simulink model "DC_Motor_project_TET41200_2"  (R2024b)
settings: Solver=ode23tb  StartTime=0.0  StopTime=5  MaxStep=10e-6  RelTol=1e-3  EnableMultiTasking=on
values from neighbouring files (symbols this model uses):
  A = 2.5    [Other_model_parameters.m]
  c_w = 0.2    [Other_model_parameters.m]
  g = 9.81    [Other_model_parameters.m]
  i_g = 10    [Other_model_parameters.m]
  J = J_car + J_m + J_g    (= 0.50375)    [Other_model_parameters.m]
  M = 2200    [Other_model_parameters.m]
  mu_r = 0.01    [Other_model_parameters.m]
  r_w = 0.25    [Other_model_parameters.m]
  rho = 1.2    [Other_model_parameters.m]
undefined symbols (not defined in the file or in its folder): DiscIntNeverNeededParam, eea_lib, PI, reg
libraries: spsVoltageMeasurementLib x8, simulink_extras x6, spsCurrentMeasurementLib x4, spsOnDelayLib x2, spsMonostableLib x2, spsControlledCurrentSourceLib x2, spsUniversalBridgeLib x2, spsDCVoltageSourceLib x1, sps_lib x1
(part 1 of 2)
settings Model: Creator=minothi  LastModifiedBy=runde
settings SolverCC: AlgebraicLoopSolver=TrustRegion  SolverResetMethod=Robust
settings DataIOCC: LimitDataPoints=on  SaveFormat=Array  SignalLoggingSaveFormat=ModelDataLogs  ReturnWorkspaceOutputs=off
settings OptimizationCC: ExpressionDepthLimit=2147483647  InitFltsAndDblsToZero=on  LifeSpan=inf
settings DebuggingCC: SaveWithParameterizedLinksMsg=none  UnderspecifiedInitializationDetection=Classic  MergeDetectMultiDrivingBlocksExec=none  SignalResolutionControl=TryResolveAllWithWarning  SolverPrmCheckMsg=warning  MultiTaskDSMMsg=warning  MultiTaskCondExecSysMsg=none  FcnCallInpInsideContextMsg=warning  UnconnectedInputMsg=warning  UnconnectedOutputMsg=warning  UnconnectedLineMsg=warning  AllowSymbolicDim=off  StateNameClashWarn=warning  SFUnexpectedBacktrackingDiag=warning  SFNoUnconditionalDefaultTransitionDiag=warning  SFExecutionAtInitializationDiag=none  ArithmeticOperatorsInVariantConditions=warning
settings HardwareCC: ProdBitPerPointer=32  ProdBitPerSizeT=32  ProdBitPerPtrDiffT=32  ProdLargestAtomicFloat=None  ProdIntDivRoundTo=Undefined  ProdEndianess=Unspecified  ProdWordSize=32  ProdHWDeviceType=32-bit Generic
settings ModelReferenceCC: EnableRefExpFcnMdlSchedulingChecks=on  PropagateSignalLabelsOutOfModel=off
settings SFSimCC: SimUseLocalCustomCode=off  CustomCodeUndefinedFunction=UseInterfaceOnly
settings RTWCC: RTWUseLocalCustomCode=off  GPUComputeCapability=3.5
settings CodeAppCC: StateflowObjectComments=on
settings GRTTargetCC: TargetFcnLib=ansi_tfl_tmw.mat  TargetLangStandard=C89/C90 (ANSI)  CombineOutputUpdateFcns=off  GRTInterface=on
settings ConfigComp: CovMetricSettings=dw  CovSaveCumulativeToWorkspaceVar=on  CovSaveSingleToWorkspaceVar=on  CovExternalEMLEnable=off
settings SimscapeCC: SimscapeNormalizeSystem=off

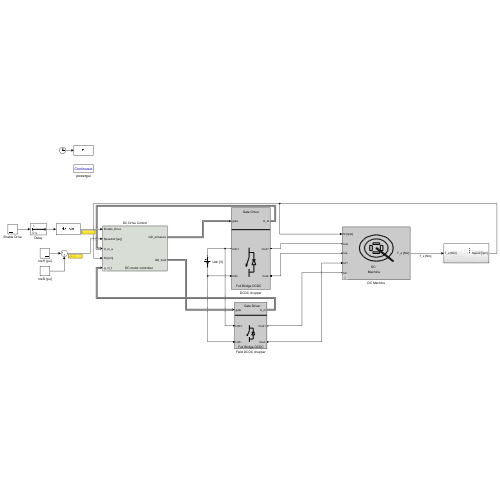
[thumbnail: Simulink's stored preview of the top-level diagram]
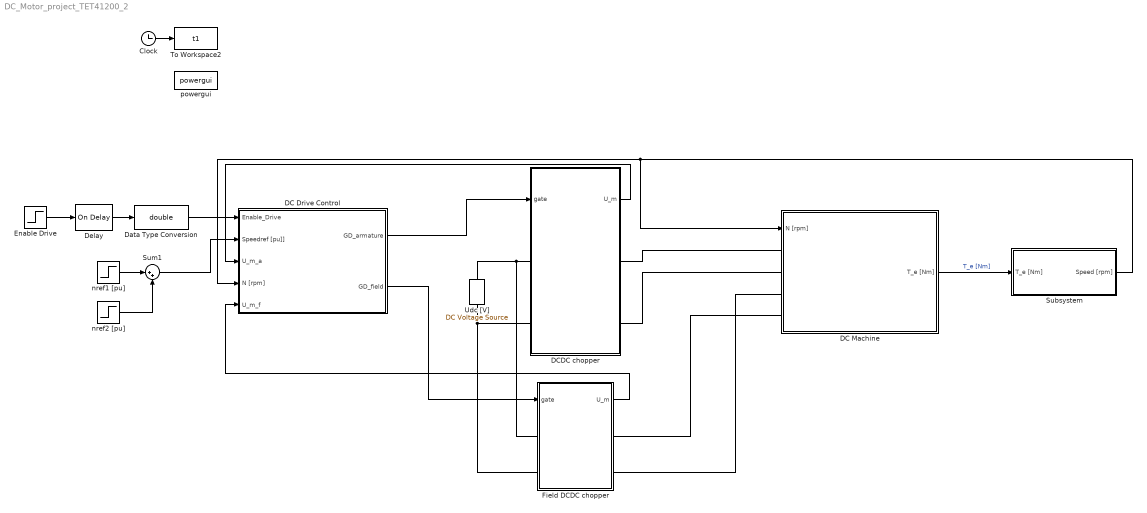
== system DC_Motor_project_TET41200_2 ==
  Clock : Clock
  DC Drive Control : Subsystem  mask{Uan=320, Ian=20, N_n=3000, Ra=1, Ufn=50, Ifn=1, I_outmax=2, I_outmin=-2, Torque_max=1.5, Torque_min=-1.5, Speed_control=1, Kp_i=0.24*1.2, Kv_i=1, Ti_i=9.75e-3, T_fa=1.0*100e-6, Kp_f=44, Ti_f=0.1, T_ff=0, Kp_n=80, Ti_n=30.8e-3, Kv_n=0, T_fn=5.5e-3, T_tri=1/1000}
      mask prompts: Uan "Uan [V]"; Ian "Ian, rated Current [A]"; N_n "Rated speed [rpm]"; Ra "Ra [Ohm]"; Ufn "Ufn [V]"; Ifn "Ifn [A]"; I_outmax "i_a,max [pu]"; I_outmin "i_a,min [pu]"; Torque_max "Torque, max [pu]"; Torque_min "Torque_min [pu]"; Speed_control "Speed control [=1. 0=Torque control]:"; Kp_i "Current controller gain K_pa"; Kv_i "Gain feedforward K__va"; Ti_i "Integration time constant T_ia"; T_fa "Armature Filter time constant T_fa [s]"; Kp_f "Field current controller gain:"; Ti_f "File Current Integration time Ti_f"; T_ff "Filter time constant field current"; Kp_n "Speed controller gain K_pn"; Ti_n "Speed Controller T_in"; Kv_n "Gain feedforward K_vn"; T_fn "Speed filter time constant"
      mask Display: text(0.350,0.08,'DC motor controller')
  DC Machine : Subsystem  mask{Uan=320, Ian=20, N_n=3000, Ra=1, La=10e-3, Ufn=50, Ifn=1, Tf=0.1}
      mask prompts: Uan "Uan, nominal Voltage [V]"; Ian "Ian, nominal current [A]"; N_n "Rated mechanical speed [rpm]"; Ra "Ra , resistance [Ohm]"; La "La,   inductance [H]"; Ufn "Ufn, nominal Field Voltage [V]"; Ifn "Ifn, nominal Field Current [A]"; Tf "Time constant field winding Tf:"
      mask Display:
      | text(0.43,0.25,'DC')
      | text(0.38,0.15,'Machine')
      | 
      | plot([0.2500    0.2600    0.2700    0.2900    0.3100    0.3300    0.3600    0.3900    0.4200    0.4600    0.5000    0.5400    0.5800    0.6100    0.6400    0.6700    0.6900    0.7100    0.7300    0.7400    0.7500], [0.6000    0.6700    0.6980    0.7356    0.7625    0.7833    0.8071    0.8245    0.8369    0.8468    0.8500    0.8468    0.8369    0.8245    0.8071    0.7833    0.7625    0.7356    0.6980    0.6700    0.6000])
      | plot([0.2500    0.2600    0.2700    0.2900    0.3100    0.3300    0.3600    0.3900    0.4200    0.4600    0.5000    0.5400    0.5800    0.6100    0.6400    0.6700    0.6900    0.7100    0.7300    0.7400    0.7500], [0.6000    0.5300    0.5020    0.4644    0.4375    0.4167    0.3929    0.3755    0.3631    0.3532    0.3500    0.3532    0.3631    0.3755    0.3929    0.4167    0.4375    0.4644    0.5020    0.5300    0.6000])
      | 
      | plot([0.3250    0.3320    0.3390    0.3530    0.3670    0.3810    0.4020    0.4230    0.4440    0.4720    0.5000    0.5280    0.5560    0.5770    0.5980    0.6190    0.6330    0.6470    0.6610    0.6680    0.6750], [0.6000    0.6490    0.6686    0.6950    0.7137    0.7283    0.7450    0.7571    0.7658    0.7727    0.7750    0.7727    0.7658    0.7571    0.7450    0.7283    0.7137    0.6950    0.6686    0.6490    0.6000])
      | plot([0.3250    0.3320    0.3390    0.3530    0.3670    0.3810    0.4020    0.4230    0.4440    0.4720    0.5000    0.5280    0.5560    0.5770    0.5980    0.6190    0.6330    0.6470    0.6610    0.6680    0.6750], [0.6000    0.5510    0.5314    0.5050    0.4863    0.4717    0.4550    0.4429    0.4342    0.4273    0.4250    0.4273    0.4342    0.4429    0.4550    0.4717    0.4863    0.5050    0.5314    0.5510    0.6000])
      | 
      | plot([0.4 0.4 0.44 0.44 0.4],   [0.55 0.65 0.65 0.55 0.55])
      | plot([0.56 0.56 0.6 0.6 0.56], [0.55 0.65 0.65 0.55 0.55])
      | plot([0.45 0.55 0.55 0.45 0.45], [0.5 0.5 0.53 0.53 0.5])
      | plot([0.45 0.55 0.55 0.45 0.45], [0.7 0.7 0.67 0.67 0.7])
      | 
      | plot([0.495 0.505 0.755 0.745 0.495], [0.595 0.605 0.355 0.345 0.595])
  DCDC chopper : Subsystem
      mask Display:
      | text(0.12,0.05,'Full Bridge DCDC')
      | text(0.3,0.95,'Gate Driver')
      | plot([0.0 1.0], [0.73 0.73])
      | plot([0.45 0.45 0.38], [0.51 0.39 0.28])
      | plot([0.45 0.45], [0.15 0.25])
      | plot([0.381 0.38 0.408], [0.317 0.28 0.302])
      | 
      | plot([0.45 0.58], [0.45 0.45])
      | plot([0.45 0.58], [0.21 0.21])
      | plot([0.58 0.58], [0.45 0.36])
      | plot([0.58 0.58], [0.21 0.30])
      | plot([0.53 0.63], [0.36 0.36])
      | plot([0.53 0.63], [0.30 0.30])
      | plot([0.53 0.58 0.63], [0.30 0.36 0.30])
  Data Type Conversion : DataTypeConversion  OutDataTypeStr=double  SaturateOnIntegerOverflow=off  RndMeth=Floor
  Delay : spsOnDelayLib/On Delay  DelayType=On delay  delay=0  ic=0  Ts=0
  Enable Drive : Step  Time=0.025  SampleTime=0
  Field DCDC chopper : Subsystem
      mask Display:
      | text(0.12,0.05,'Full Bridge DCDC')
      | text(0.3,0.95,'Gate Driver')
      | plot([0.0 1.0], [0.73 0.73])
      | plot([0.45 0.45 0.38], [0.51 0.39 0.28])
      | plot([0.45 0.45], [0.15 0.25])
      | plot([0.381 0.38 0.408], [0.317 0.28 0.302])
      | 
      | plot([0.45 0.58], [0.45 0.45])
      | plot([0.45 0.58], [0.21 0.21])
      | plot([0.58 0.58], [0.45 0.36])
      | plot([0.58 0.58], [0.21 0.30])
      | plot([0.53 0.63], [0.36 0.36])
      | plot([0.53 0.63], [0.30 0.30])
      | plot([0.53 0.58 0.63], [0.30 0.36 0.30])
  Subsystem : Subsystem
  Sum1 : Sum  Inputs=|++
  To Workspace2 : ToWorkspace  VariableName=t1  SampleTime=1e-3
  Udc [V] : spsDCVoltageSourceLib/DC Voltage Source  Amplitude=360  Measurements=None
  nref1 [pu] : Step  Time=0.2  After=-5  SampleTime=0
  nref2 [pu] : Step  Time=0.9  After=-0.1  SampleTime=0
  powergui : sps_lib/powergui  SimulationMode=Continuous  SampleTime=0  frequency=60  Iterations=50  frequencyindice=0  Pbase=100e6  ErrMax=1e-4  UnitsV=kV  UnitsW=MW  buscounter=0  FunctionMessages=off  echomessages=off  EnableUseOfTLC=off  CurrentSourceSwitches=on  DisableSnubberDevices=off  DisableRonSwitches=off  DisableVfSwitches=off  DisplayEquations=off  AutomaticDiscreteSolvers=off  SolverType=Tustin  Interpol=off  ExternalGateDelay=off  methode=off  Ts=0  x0status=blocks  SPID=off  SwTol=0  HookPort=off  NonlinearTolerance=1e-4  nMaxIteration=100  ContinueOnMaxIteration=off  RestoreLinks=warning  ResistiveCurrentMeasurement=off  Frange=[0:2:500]  Ylog=off  Xlog=on  ShowGrid=off  save=off  variable=ZData  structure=0  ZoomFFT=on  StartTime=0.0  cycles=1  DisplayStyle=1  fundamental=60  FreqAxis=off  MaxFrequency=1000  frequencyindicesteady=1  RmsSteady=1  display=off
  wires:
  Clock/1 -> To Workspace2/1
  Enable Drive/1 -> Delay/1
  DCDC chopper/1(" U_m") -> DC Drive Control/3(U_m_a)
  DC Drive Control/1(GD_armature) -> DCDC chopper/1(gate)
  Delay/1 -> Data Type Conversion/1
  Data Type Conversion/1 -> DC Drive Control/1(Enable_Drive)
  nref1 [pu]/1 -> Sum1/1
  nref2 [pu]/1 -> Sum1/2
  Sum1/1 -> DC Drive Control/2(Speedref [pu]])
  DC Drive Control/2(GD_field) -> Field DCDC chopper/1(gate)
  Field DCDC chopper/1(" U_m") -> DC Drive Control/5(U_m_f)
  Subsystem/1(Speed [rpm]) -> DC Drive Control/4(N [rpm]), DC Machine/1(N [rpm])
  DC Machine/1(T_e [Nm]) -> Subsystem/1(T_e [Nm])  "T_e [Nm]"
  connections:
  Udc [V]/RConn1 -- Field DCDC chopper/LConn1 -- DCDC chopper/LConn1
  Udc [V]/LConn1 -- DCDC chopper/LConn2 -- Field DCDC chopper/LConn2
  DC Machine/LConn1 -- DCDC chopper/RConn1
  DC Machine/LConn2 -- DCDC chopper/RConn2
  Field DCDC chopper/RConn2 -- DC Machine/LConn3
  DC Machine/LConn4 -- Field DCDC chopper/RConn1

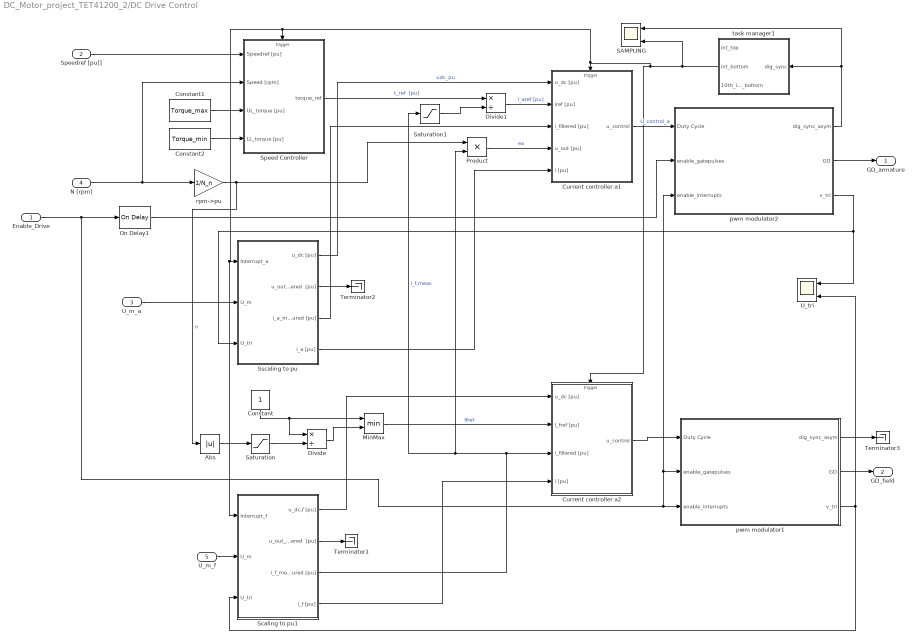
== system DC_Motor_project_TET41200_2/DC Drive Control ==
  Enable_Drive : Inport
  Speedref [pu]] : Inport  Port=2
  U_m_a : Inport  Port=3
  N [rpm] : Inport  Port=4
  U_m_f : Inport  Port=5
  Abs : Abs  SaturateOnIntegerOverflow=off
  Constant : Constant
  Constant1 : Constant  Value=Torque_max
  Constant2 : Constant  Value=Torque_min
  Current controller a1 : Subsystem
  Current controller a2 : Subsystem
  Divide : Product  Inputs=*/
  Divide1 : Product  Inputs=*/
  MinMax : MinMax  Inputs=2
  On Delay1 : spsOnDelayLib/On Delay  DelayType=On delay  delay=0  ic=0  Ts=0
  Product : Product
  SAMPLING : Scope  NumInputPorts=2
  Saturation : Saturate  UpperLimit=Inf  LowerLimit=0.01
  Saturation1 : Saturate  UpperLimit=Inf  LowerLimit=0.01
  Scaling to pu1 : Subsystem
  Speed Controller : Subsystem
  Sscaling to pu : Subsystem
  Terminator1 : Terminator
  Terminator2 : Terminator
  Terminator3 : Terminator
  U_tri : Scope  NumInputPorts=2
  pwm modulator1 : Subsystem  mask{T_tri=T_tri, t_dead=1.0e-6, t_min=3.0e-6, type_signal=1, asym=on}
      mask prompts: T_tri "Switching period  [sec]"; t_dead "t_dead, blanking time for the switches"; t_min "t_min, minimum turn off time for the swtches"; type_signal "type_signal, type of reference voltage signal (1 or 2)"; asym "Asymmetrical PWM"
      mask help:
      | The pwm module simulates a three-phase pulse-width modulator and sets the digital switch signals for six inverter switches. Nonlinear effects as blanking time and minimum turn-off time is implemented.
      |
      | As reference voltage signal can one of the following be chosen:
      | 1 - pure sinus
      | 2 - sinus with the injection of the third harmonic
      mask Display:
      | text(0.38,0.2,'DC asym pwm')
      | 
      | plot([0.32 0.32 0.68 0.68 0.32], [0.4 0.8 0.8 0.4 0.4])
      | plot([0.34 0.38 0.42 0.46 0.50 0.54 0.58 0.62 0.66], [0.5 0.7 0.5 0.7 0.5 0.7 0.5 0.7 0.5])
      | plot([0.3400    0.3600    0.3800    0.4000    0.4200    0.4400    0.4600    0.4800    0.5000    0.5200    0.5400    0.5600    0.5800    0.6000    0.6200    0.6400    0.6600], [0.6053    0.5699    0.5392    0.5182    0.5100    0.5161    0.5354    0.5650    0.6000    0.6350    0.6646    0.6839    0.6900    0.6818    0.6608    0.6301    0.5947])
  pwm modulator2 : Subsystem  mask{T_tri=T_tri, t_dead=1.0e-6, t_min=3.0e-6, type_signal=1, asym=on}
      mask prompts: T_tri "Switching period  [sec]"; t_dead "t_dead, blanking time for the switches"; t_min "t_min, minimum turn off time for the swtches"; type_signal "type_signal, type of reference voltage signal (1 or 2)"; asym "Asymmetrical PWM"
      mask help:
      | The pwm module simulates a three-phase pulse-width modulator and sets the digital switch signals for six inverter switches. Nonlinear effects as blanking time and minimum turn-off time is implemented.
      |
      | As reference voltage signal can one of the following be chosen:
      | 1 - pure sinus
      | 2 - sinus with the injection of the third harmonic
      mask Display:
      | text(0.38,0.2,'DC asym pwm')
      | 
      | plot([0.32 0.32 0.68 0.68 0.32], [0.4 0.8 0.8 0.4 0.4])
      | plot([0.34 0.38 0.42 0.46 0.50 0.54 0.58 0.62 0.66], [0.5 0.7 0.5 0.7 0.5 0.7 0.5 0.7 0.5])
      | plot([0.3400    0.3600    0.3800    0.4000    0.4200    0.4400    0.4600    0.4800    0.5000    0.5200    0.5400    0.5600    0.5800    0.6000    0.6200    0.6400    0.6600], [0.6053    0.5699    0.5392    0.5182    0.5100    0.5161    0.5354    0.5650    0.6000    0.6350    0.6646    0.6839    0.6900    0.6818    0.6608    0.6301    0.5947])
  rpm->pu : Gain  Gain=1/N_n
  task manager1 : Subsystem  mask{T_exec_0=20e-6}
      mask prompts: T_exec_0 "Execution time of Int0 (less than 0.5 T_tri)"
  GD_armature : Outport
  GD_field : Outport  Port=2
  wires:
  U_m_a/1 -> Sscaling to pu/2(U_m)
  Enable_Drive/1 -> pwm modulator1/3(enable_interrupts), pwm modulator1/2(enable_gatepulses), pwm modulator2/3(enable_interrupts), On Delay1/1
  Speed Controller/1(torque_ref) -> Divide1/1  "t_ref  [pu]"
  Sscaling to pu/3(i_a_mesured [pu]) -> Current controller a1/3(i_filtered [pu])
  Sscaling to pu/1(u_dc [pu]) -> Current controller a1/1(u_dc [pu])  "udc_pu"
  Current controller a1/1(u_control) -> pwm modulator2/1(Duty Cycle)  "U_control_a"
  N [rpm]/1 -> rpm->pu/1, Speed Controller/2(Speed [rpm])
  rpm->pu/1 -> Product/1, Abs/1  "n"
  Sscaling to pu/2(u_out_filtered  [pu]) -> Terminator2/1
  Sscaling to pu/4(i_a [pu]) -> Current controller a1/5(i [pu])
  Speedref [pu]]/1 -> Speed Controller/1(Speedref [pu])
  On Delay1/1 -> pwm modulator2/2(enable_gatepulses)
  U_m_f/1 -> Scaling to pu1/2(U_m)
  Scaling to pu1/3(i_f_mesured [pu]) -> Product/2, Saturation1/1, Current controller a2/3(i_filtered [pu])  "i_f,meas"
  Scaling to pu1/1(u_dc,f [pu]) -> Current controller a2/1(u_dc [pu])
  Constant/1 -> MinMax/1, Divide/1
  Abs/1 -> Saturation/1
  Saturation/1 -> Divide/2
  Divide/1 -> MinMax/2
  MinMax/1 -> Current controller a2/2(i_fref [pu])  "Ifref"
  Saturation1/1 -> Divide1/2
  Divide1/1 -> Current controller a1/2(iref [pu])  "i_aref [pu]"
  pwm modulator2/2(GD) -> GD_armature/1
  pwm modulator1/2(GD) -> GD_field/1
  pwm modulator2/1(dig_sync_asym) -> SAMPLING/1, task manager1/1(dig_sync)
  task manager1/2(int_bottom) -> SAMPLING/2, Current controller a2/Trigger, Speed Controller/Trigger, Scaling to pu1/1(Interrupt_f), Sscaling to pu/1(Interrupt_a), Current controller a1/Trigger
  pwm modulator1/3(v_tri) -> Scaling to pu1/3(U_tri), U_tri/2
  pwm modulator1/1(dig_sync_asym) -> Terminator3/1
  pwm modulator2/3(v_tri) -> U_tri/1, Sscaling to pu/3(U_tri)
  Current controller a2/1(u_control) -> pwm modulator1/1(Duty Cycle)
  Product/1 -> Current controller a1/4(u_out [pu])  "ea"
  Scaling to pu1/4(i_f [pu]) -> Current controller a2/4(i [pu])
  Scaling to pu1/2(u_out_filtered  [pu]) -> Terminator1/1
  Constant1/1 -> Speed Controller/3(UL_torque [pu])
  Constant2/1 -> Speed Controller/4(LL_torque [pu])

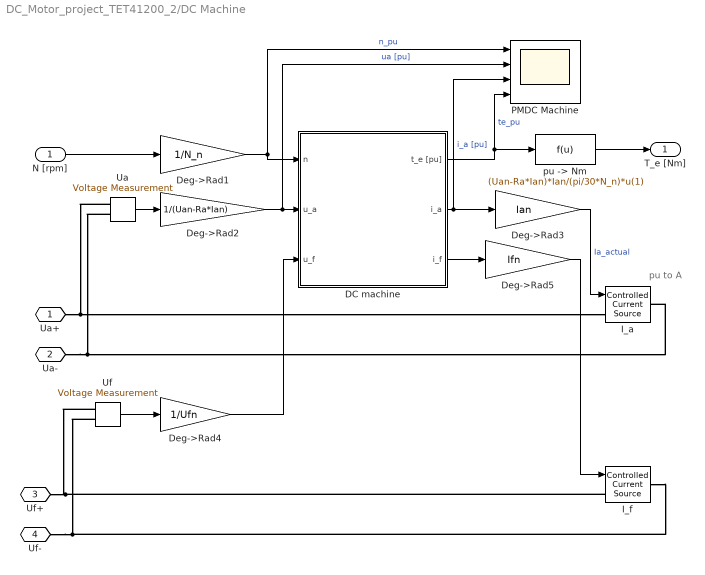
== system DC_Motor_project_TET41200_2/DC Machine ==
  note: pu to A
  N [rpm] : Inport
  DC machine : Subsystem  mask{r_a=Ra*Ian/(Uan-Ra*Ian), l_a=La*Ian/(Uan-Ra*Ian), T_f=Tf}
      mask prompts: r_a "r_a in [p.u.]"; l_a "l_a in [p.u]"; T_f "Field time constant Tf :"
      mask Display: text(0.32,0.9,'DC')
  Deg->Rad1 : Gain  Gain=1/N_n  SaturateOnIntegerOverflow=on  OutDataTypeStr=Inherit: Same as input  ParamDataTypeStr=Inherit: Same as input
  Deg->Rad2 : Gain  Gain=1/(Uan-Ra*Ian)  SaturateOnIntegerOverflow=on  OutDataTypeStr=Inherit: Same as input  ParamDataTypeStr=Inherit: Same as input
  Deg->Rad3 : Gain  Gain=Ian  SaturateOnIntegerOverflow=on  OutDataTypeStr=Inherit: Same as input  ParamDataTypeStr=Inherit: Same as input
  Deg->Rad4 : Gain  Gain=1/Ufn  SaturateOnIntegerOverflow=on  OutDataTypeStr=Inherit: Same as input  ParamDataTypeStr=Inherit: Same as input
  Deg->Rad5 : Gain  Gain=Ifn  SaturateOnIntegerOverflow=on  OutDataTypeStr=Inherit: Same as input  ParamDataTypeStr=Inherit: Same as input
  I_a : spsControlledCurrentSourceLib/Controlled Current Source  Initialize=on  Source_Type=AC  Amplitude=0  Phase=0  Frequency=0  Measurements=None
  I_f : spsControlledCurrentSourceLib/Controlled Current Source  Initialize=on  Source_Type=AC  Amplitude=0  Phase=0  Frequency=0  Measurements=None
  PMDC Machine : Scope  NumInputPorts=4
  Ua : spsVoltageMeasurementLib/Voltage Measurement  PhasorSimulation=off  OutputType=Complex  PSBequivalent=0
  Uf : spsVoltageMeasurementLib/Voltage Measurement  PhasorSimulation=off  OutputType=Complex  PSBequivalent=0
  "pu -> Nm" : Fcn  Expr=(Uan-Ra*Ian)*Ian/(pi/30*N_n)*u(1)
  Ua+ : PMIOPort  Side=Left
  Ua- : PMIOPort  Port=2  Side=Left
  Uf+ : PMIOPort  Port=3  Side=Left
  Uf- : PMIOPort  Port=4  Side=Left
  T_e [Nm] : Outport  InitialOutput=0
  wires:
  Deg->Rad2/1 -> PMDC Machine/2, DC machine/2(u_a)  "ua [pu]"
  Deg->Rad3/1 -> I_a/1  "Ia_actual"
  DC machine/2(i_a) -> Deg->Rad3/1, PMDC Machine/3  "i_a [pu]"
  Deg->Rad1/1 -> PMDC Machine/1, DC machine/1(n)  "n_pu"
  N [rpm]/1 -> Deg->Rad1/1
  Ua/1 -> Deg->Rad2/1
  "pu -> Nm"/1 -> T_e [Nm]/1
  DC machine/1(t_e [pu]) -> PMDC Machine/4, "pu -> Nm"/1  "te_pu"
  Uf/1 -> Deg->Rad4/1
  Deg->Rad4/1 -> DC machine/3(u_f)
  DC machine/3(i_f) -> Deg->Rad5/1
  Deg->Rad5/1 -> I_f/1
  connections:
  Ua-/RConn1 -- Ua/LConn2 -- I_a/RConn1
  Ua+/RConn1 -- Ua/LConn1 -- I_a/LConn1
  Uf/LConn1 -- I_f/LConn1 -- Uf+/RConn1
  Uf/LConn2 -- I_f/RConn1 -- Uf-/RConn1

== system DC_Motor_project_TET41200_2/DCDC chopper ==
  gate : Inport
  Armarture Converter currents : Scope  NumInputPorts=2
  Armarture Converter currents1 : Scope  NumInputPorts=2
  Demux : Demux  Outputs=2
  Idc : spsCurrentMeasurementLib/Current Measurement  PhasorSimulation=off  OutputType=Complex  PSBequivalent=0
  Iout : spsCurrentMeasurementLib/Current Measurement  PhasorSimulation=off  OutputType=Complex  PSBequivalent=0
  Universal Bridge : spsUniversalBridgeLib/Universal Bridge  Arms=2  SnubberResistance=1e5  SnubberCapacitance=inf  Device=MOSFET / Diodes  Ron=1e-3  Lon=0  ForwardVoltages="[  0  0  ]"  ForwardVoltage=0  GTOparameters=[ 10e-6 , 20e-6 ]  IGBTparameters=[ 1e-6 , 2e-6 ]  Measurements=All voltages and currents  Measurements_2=None  converterType=Rectifier
  u_m : Subsystem
  Udc+ : PMIOPort  Side=Left
  Udc- : PMIOPort  Port=2  Side=Left
  Vout+ : PMIOPort  Port=3  Side=Right
  Vout- : PMIOPort  Port=4  Side=Right
  " U_m" : Outport
  wires:
  u_m/1(U) -> " U_m"/1
  gate/1 -> Demux/1, Universal Bridge/1
  Iout/1 -> Armarture Converter currents/1, u_m/1(Ia)  "I_Out [A]"
  Idc/1 -> Armarture Converter currents/2  "i_DC [A]"
  Demux/2 -> Armarture Converter currents1/2
  Demux/1 -> Armarture Converter currents1/1
  connections:
  Universal Bridge/LConn1 -- Iout/LConn1
  Idc/LConn1 -- Udc+/RConn1
  Udc-/RConn1 -- u_m/LConn2 -- Universal Bridge/RConn2
  Universal Bridge/RConn1 -- u_m/LConn1 -- Idc/RConn1
  Vout+/RConn1 -- Iout/RConn1
  u_m/LConn4 -- Universal Bridge/LConn2 -- u_m/LConn3 -- Vout-/RConn1

== system DC_Motor_project_TET41200_2/Field DCDC chopper ==
  gate : Inport
  Field Converter currents : Scope  NumInputPorts=2
  Idc : spsCurrentMeasurementLib/Current Measurement  PhasorSimulation=off  OutputType=Complex  PSBequivalent=0
  Iout : spsCurrentMeasurementLib/Current Measurement  PhasorSimulation=off  OutputType=Complex  PSBequivalent=0
  Universal Bridge : spsUniversalBridgeLib/Universal Bridge  Arms=2  SnubberResistance=1e5  SnubberCapacitance=inf  Device=MOSFET / Diodes  Ron=1e-3  Lon=0  ForwardVoltages="[  0  0  ]"  ForwardVoltage=0  GTOparameters=[ 10e-6 , 20e-6 ]  IGBTparameters=[ 1e-6 , 2e-6 ]  Measurements=All voltages and currents  Measurements_2=None  converterType=Rectifier
  u_m : Subsystem
  Udc+ : PMIOPort  Side=Left
  Udc- : PMIOPort  Port=2  Side=Left
  Vout+ : PMIOPort  Port=3  Side=Right
  Vout- : PMIOPort  Port=4  Side=Right
  " U_m" : Outport
  wires:
  u_m/1(U) -> " U_m"/1
  gate/1 -> Universal Bridge/1
  Iout/1 -> Field Converter currents/1, u_m/1(Ia)  "I_Out [A]"
  Idc/1 -> Field Converter currents/2  "i_DC [A]"
  connections:
  Vout-/RConn1 -- Universal Bridge/LConn2 -- u_m/LConn4
  Idc/LConn1 -- Udc+/RConn1
  Udc-/RConn1 -- u_m/LConn2 -- Universal Bridge/RConn2
  Universal Bridge/RConn1 -- u_m/LConn1 -- Idc/RConn1
  Vout+/RConn1 -- Iout/RConn1
  Universal Bridge/LConn1 -- Iout/LConn1 -- u_m/LConn3

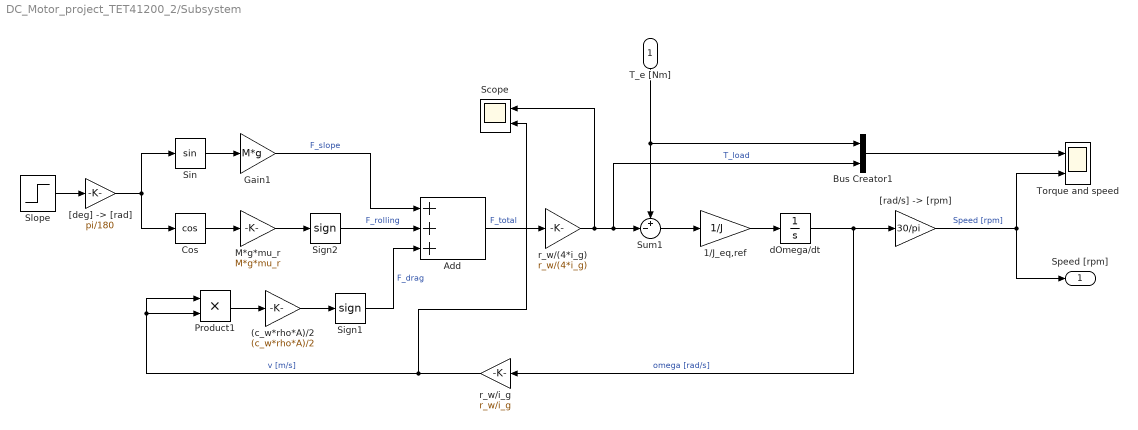
== system DC_Motor_project_TET41200_2/Subsystem ==
  T_e [Nm] : Inport
  (c_w*rho*A)/2 : Gain  Gain=(c_w*rho*A)/2
  1/J_eq,ref : Gain  Gain=1/J
  Add : Sum  Inputs=+++
  Bus Creator1 : BusCreator  Inputs=2
  Cos : Trigonometry  Operator=cos
  Gain1 : Gain  Gain=M*g
  M*g*mu_r : Gain  Gain=M*g*mu_r
  Product1 : Product
  Scope : Scope  NumInputPorts=2
  Sign1 : Signum
  Sign2 : Signum
  Sin : Trigonometry
  Slope : Step  Time=0.4  After=0  SampleTime=0
  Sum1 : Sum  Inputs=+-|
  Torque and speed : Scope  NumInputPorts=2
  "[deg] -> [rad]" : Gain  Gain=pi/180
  "[rad/s] -> [rpm]" : Gain  Gain=30/pi
  dOmega/dt : Integrator
  r_w/(4*i_g) : Gain  Gain=r_w/(4*i_g)
  r_w/i_g : Gain  Gain=r_w/i_g
  Speed [rpm] : Outport
  wires:
  Add/1 -> r_w/(4*i_g)/1  "F_total"
  1/J_eq,ref/1 -> dOmega/dt/1
  T_e [Nm]/1 -> Sum1/1, Bus Creator1/1
  Sin/1 -> Gain1/1
  Slope/1 -> "[deg] -> [rad]"/1
  Sign1/1 -> Add/3  "F_drag"
  Gain1/1 -> Add/1  "F_slope"
  Product1/1 -> (c_w*rho*A)/2/1
  r_w/(4*i_g)/1 -> Scope/1, Bus Creator1/2, Sum1/2  "T_load"
  Sign2/1 -> Add/2  "F_rolling"
  Bus Creator1/1 -> Torque and speed/1
  M*g*mu_r/1 -> Sign2/1
  Cos/1 -> M*g*mu_r/1
  Sum1/1 -> 1/J_eq,ref/1
  r_w/i_g/1 -> Scope/2, Product1/1, Product1/2  "v [m/s]"
  "[rad/s] -> [rpm]"/1 -> Speed [rpm]/1, Torque and speed/2  "Speed [rpm]"
  (c_w*rho*A)/2/1 -> Sign1/1
  dOmega/dt/1 -> "[rad/s] -> [rpm]"/1, r_w/i_g/1  "omega [rad/s]"
  "[deg] -> [rad]"/1 -> Sin/1, Cos/1

== system DC_Motor_project_TET41200_2/DC Drive Control/Current controller a1 ==
  u_dc [pu] : Inport
  iref [pu] : Inport  Port=2
  i_filtered [pu] : Inport  Port=3
  u_out [pu] : Inport  Port=4
  i [pu] : Inport  Port=5
  Trigger : TriggerPort  VariantControl=Variant
  "Armature Current Controller " : Scope  NumInputPorts=2
  Bus Creator : BusCreator  Inputs=3
  Constant : Constant
  Constant1 : Constant  Value=-1
  Current controller a : Subsystem  AncestorBlock=eea_lib/PI-reg  TreatAsAtomicUnit=on  mask{Kp=0.03, Kv=Kv_i, Ti=Ti_i, Tsamp=T_tri/2}
      mask Display:
      | text(0.32,0.05,'Digital PI-controller')
      | plot([0.2 0.8], [0.1 0.1])
      | plot([0.2 0.2], [0.1 0.9])
      | plot([0.75 0.8 0.75], [0.15 0.1 0.05])
      | plot([0.175 0.2 0.225], [0.79 0.9 0.79])
      | 
      | plot([0.2 0.75], [0.3 0.7])
  Sum : Sum  Inputs=|+-
  u_control : Outport
  wires:
  Constant1/1 -> Current controller a/5(LL)
  u_out [pu]/1 -> Current controller a/3(back_emf), Current controller a/6(Initival)
  Constant/1 -> Current controller a/4(UL)
  Sum/1 -> Current controller a/2(e)
  Bus Creator/1 -> "Armature Current Controller "/1
  Current controller a/1(Out) -> "Armature Current Controller "/2, u_control/1  "u_control"
  i [pu]/1 -> Bus Creator/3  "i_a [pu]"
  iref [pu]/1 -> Sum/1, Bus Creator/1  "i_aref [pu]"
  u_dc [pu]/1 -> Current controller a/1(gain)
  i_filtered [pu]/1 -> Bus Creator/2, Sum/2  "i_a_filtered [pu]"

== system DC_Motor_project_TET41200_2/DC Drive Control/Current controller a2 ==
  u_dc [pu] : Inport
  i_fref [pu] : Inport  Port=2
  i_filtered [pu] : Inport  Port=3
  i [pu] : Inport  Port=4
  Trigger : TriggerPort  VariantControl=Variant
  Bus Creator : BusCreator  Inputs=3
  Constant : Constant  Value=1.0
  Constant1 : Constant  Value=-1.0
  Current controller f : Subsystem  AncestorBlock=eea_lib/PI-reg  TreatAsAtomicUnit=on  mask{Kp=100, Kv=0, Ti=Ti_f, Tsamp=T_tri/2}
      mask Display:
      | text(0.32,0.05,'Digital PI-controller')
      | plot([0.2 0.8], [0.1 0.1])
      | plot([0.2 0.2], [0.1 0.9])
      | plot([0.75 0.8 0.75], [0.15 0.1 0.05])
      | plot([0.175 0.2 0.225], [0.79 0.9 0.79])
      | 
      | plot([0.2 0.75], [0.3 0.7])
  "Field Current Controller " : Scope  NumInputPorts=2
  Sum : Sum  Inputs=|+-
  u_control : Outport
  wires:
  Constant1/1 -> Current controller f/4(LL)
  Constant/1 -> Current controller f/3(UL)
  Sum/1 -> Current controller f/2(e)
  Bus Creator/1 -> "Field Current Controller "/1
  Current controller f/1(Out) -> "Field Current Controller "/2, u_control/1  "u_control_f"
  i [pu]/1 -> Bus Creator/3  "i_f [pu]"
  i_fref [pu]/1 -> Bus Creator/1, Sum/1  "i_fref [pu]"
  u_dc [pu]/1 -> Current controller f/1(gain)
  i_filtered [pu]/1 -> Sum/2, Bus Creator/2  "i_f_filtered [pu]"

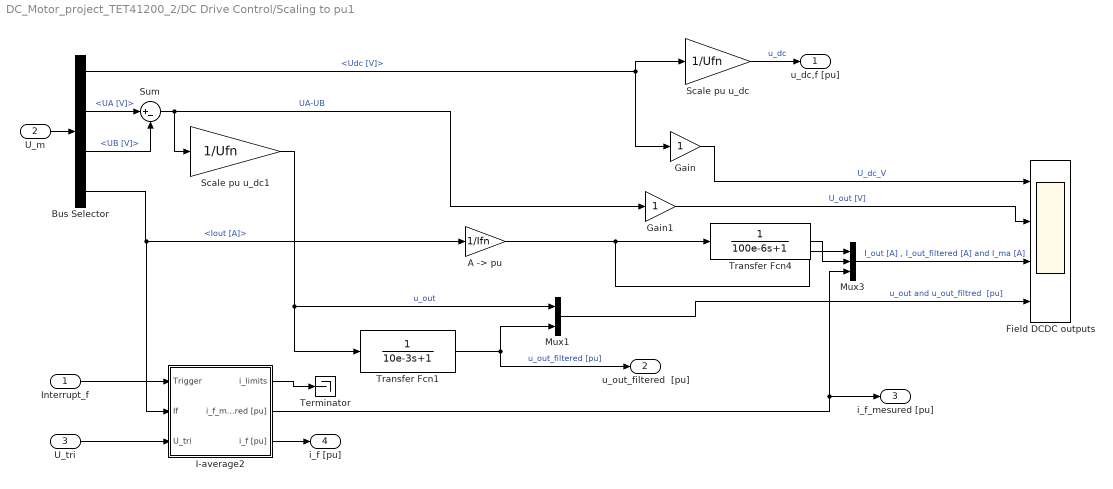
== system DC_Motor_project_TET41200_2/DC Drive Control/Scaling to pu1 ==
  Interrupt_f : Inport
  U_m : Inport  Port=2
  U_tri : Inport  Port=3
  "A -> pu" : Gain  Gain=1/Ifn
  Bus Selector : BusSelector  OutputSignals=Udc [V],UA [V],UB [V],Iout [A]
  Field DCDC outputs : Scope  NumInputPorts=4
  Gain : Gain
  Gain1 : Gain
  I-average2 : Subsystem  mask{Tsamp=T_tri/2}
  Mux1 : Mux  Inputs=2
  Mux3 : Mux  Inputs=3
  Scale pu u_dc : Gain  Gain=1/Ufn
  Scale pu u_dc1 : Gain  Gain=1/Ufn
  Sum : Sum  Inputs=|+-
  Terminator : Terminator
  Transfer Fcn1 : TransferFcn  Denominator=[10e-3 1]
  Transfer Fcn4 : TransferFcn  Denominator=[100e-6 1]
  u_dc,f [pu] : Outport
  u_out_filtered  [pu] : Outport  Port=2
  i_f_mesured [pu] : Outport  Port=3
  i_f [pu] : Outport  Port=4
  wires:
  Scale pu u_dc/1 -> u_dc,f [pu]/1  "u_dc"
  U_m/1 -> Bus Selector/1
  Scale pu u_dc1/1 -> Transfer Fcn1/1, Mux1/1  "u_out"
  Bus Selector/1 -> Scale pu u_dc/1, Gain/1  "<Udc [V]>"
  Gain/1 -> Field DCDC outputs/1  "U_dc_V"
  Bus Selector/2 -> Sum/1  "<UA [V]>"
  Gain1/1 -> Field DCDC outputs/2  "U_out [V]"
  Bus Selector/4 -> "A -> pu"/1, I-average2/2(If)  "<Iout [A]>"
  Transfer Fcn1/1 -> Mux1/2, u_out_filtered  [pu]/1  "u_out_filtered [pu]"
  Mux1/1 -> Field DCDC outputs/4  "u_out and u_out_filtred  [pu]"
  Transfer Fcn4/1 -> Mux3/2
  Mux3/1 -> Field DCDC outputs/3  "I_out [A] , I_out_filtered [A] and I_ma [A]"
  Interrupt_f/1 -> I-average2/1(Trigger)
  I-average2/2(i_f_measured [pu]) -> i_f_mesured [pu]/1, Mux3/3
  I-average2/1(i_limits) -> Terminator/1
  Bus Selector/3 -> Sum/2  "<UB [V]>"
  Sum/1 -> Scale pu u_dc1/1, Gain1/1  "UA-UB"
  I-average2/3(i_f [pu]) -> i_f [pu]/1
  U_tri/1 -> I-average2/3(U_tri)
  "A -> pu"/1 -> Transfer Fcn4/1, Mux3/1

== system DC_Motor_project_TET41200_2/DC Drive Control/Speed Controller ==
  Speedref [pu] : Inport
  Speed [rpm] : Inport  Port=2
  UL_torque [pu] : Inport  Port=3
  LL_torque [pu] : Inport  Port=4
  Trigger : TriggerPort  VariantControl=Variant
  1st order Discrete Filter : DiscreteFilter  Numerator=[T_tri/(2*T_fn)]  Denominator=[1 -(1-T_tri/(2*T_fn))]
  Bus Creator : BusCreator  Inputs=3
  "Speed Controller Controller " : Scope  NumInputPorts=3
  "Speed controller " : Subsystem  AncestorBlock=eea_lib/PI-reg  TreatAsAtomicUnit=on  mask{Kp=Kp_n, Kv=Kv_n, Ti=Ti_n, Tsamp=T_tri/2}
      mask Display:
      | text(0.32,0.05,'Digital PI-controller')
      | plot([0.2 0.8], [0.1 0.1])
      | plot([0.2 0.2], [0.1 0.9])
      | plot([0.75 0.8 0.75], [0.15 0.1 0.05])
      | plot([0.175 0.2 0.225], [0.79 0.9 0.79])
      | 
      | plot([0.2 0.75], [0.3 0.7])
  Sum : Sum  Inputs=|+-
  rpm->pu : Gain  Gain=1/N_n
  torque_ref : Outport
  wires:
  Sum/1 -> "Speed controller "/1(e), "Speed Controller Controller "/2  "n_ref - n_filtered [pu]"
  Speedref [pu]/1 -> Sum/1, Bus Creator/1  "n_ref [pu]"
  rpm->pu/1 -> 1st order Discrete Filter/1, Sum/2, Bus Creator/3  "n  [pu]"
  Speed [rpm]/1 -> rpm->pu/1
  Bus Creator/1 -> "Speed Controller Controller "/1
  "Speed controller "/1(Out) -> "Speed Controller Controller "/3, torque_ref/1
  UL_torque [pu]/1 -> "Speed controller "/2(UL)
  LL_torque [pu]/1 -> "Speed controller "/3(LL)
  1st order Discrete Filter/1 -> Bus Creator/2  "n_filtered [pu]"

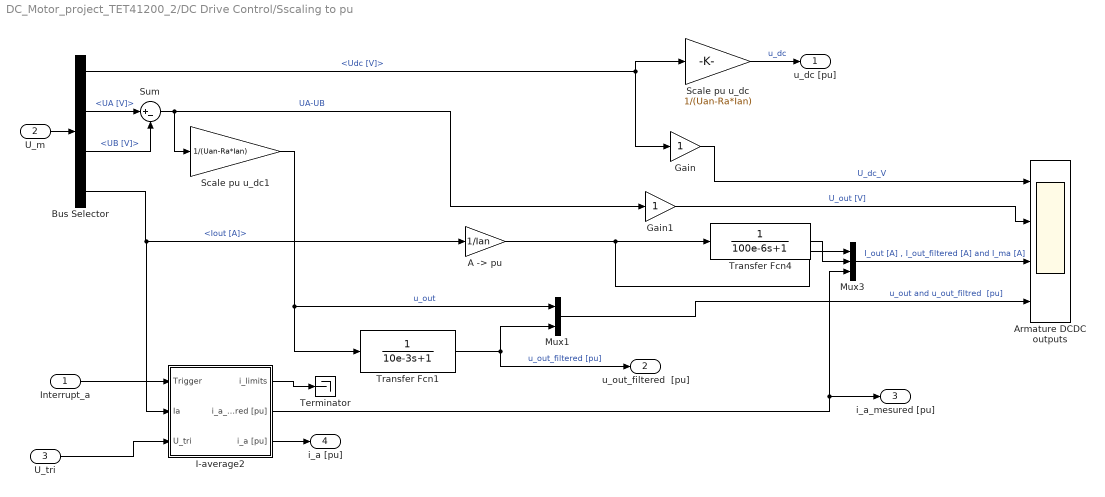
== system DC_Motor_project_TET41200_2/DC Drive Control/Sscaling to pu ==
  Interrupt_a : Inport
  U_m : Inport  Port=2
  U_tri : Inport  Port=3
  "A -> pu" : Gain  Gain=1/Ian
  Armature DCDC outputs : Scope  NumInputPorts=4
  Bus Selector : BusSelector  OutputSignals=Udc [V],UA [V],UB [V],Iout [A]
  Gain : Gain
  Gain1 : Gain
  I-average2 : Subsystem  mask{Tsamp=T_tri/2}
  Mux1 : Mux  Inputs=2
  Mux3 : Mux  Inputs=3
  Scale pu u_dc : Gain  Gain=1/(Uan-Ra*Ian)
  Scale pu u_dc1 : Gain  Gain=1/(Uan-Ra*Ian)
  Sum : Sum  Inputs=|+-
  Terminator : Terminator
  Transfer Fcn1 : TransferFcn  Denominator=[10e-3 1]
  Transfer Fcn4 : TransferFcn  Denominator=[100e-6 1]
  u_dc [pu] : Outport
  u_out_filtered  [pu] : Outport  Port=2
  i_a_mesured [pu] : Outport  Port=3
  i_a [pu] : Outport  Port=4
  wires:
  Scale pu u_dc/1 -> u_dc [pu]/1  "u_dc"
  U_m/1 -> Bus Selector/1
  Scale pu u_dc1/1 -> Transfer Fcn1/1, Mux1/1  "u_out"
  Bus Selector/1 -> Scale pu u_dc/1, Gain/1  "<Udc [V]>"
  Gain/1 -> Armature DCDC outputs/1  "U_dc_V"
  Bus Selector/2 -> Sum/1  "<UA [V]>"
  Gain1/1 -> Armature DCDC outputs/2  "U_out [V]"
  Bus Selector/4 -> "A -> pu"/1, I-average2/2(Ia)  "<Iout [A]>"
  Transfer Fcn1/1 -> Mux1/2, u_out_filtered  [pu]/1  "u_out_filtered [pu]"
  Mux1/1 -> Armature DCDC outputs/4  "u_out and u_out_filtred  [pu]"
  Transfer Fcn4/1 -> Mux3/2
  Mux3/1 -> Armature DCDC outputs/3  "I_out [A] , I_out_filtered [A] and I_ma [A]"
  Interrupt_a/1 -> I-average2/1(Trigger)
  I-average2/2(i_a_measured [pu]) -> i_a_mesured [pu]/1, Mux3/3
  I-average2/1(i_limits) -> Terminator/1
  Bus Selector/3 -> Sum/2  "<UB [V]>"
  Sum/1 -> Scale pu u_dc1/1, Gain1/1  "UA-UB"
  I-average2/3(i_a [pu]) -> i_a [pu]/1
  U_tri/1 -> I-average2/3(U_tri)
  "A -> pu"/1 -> Transfer Fcn4/1, Mux3/1

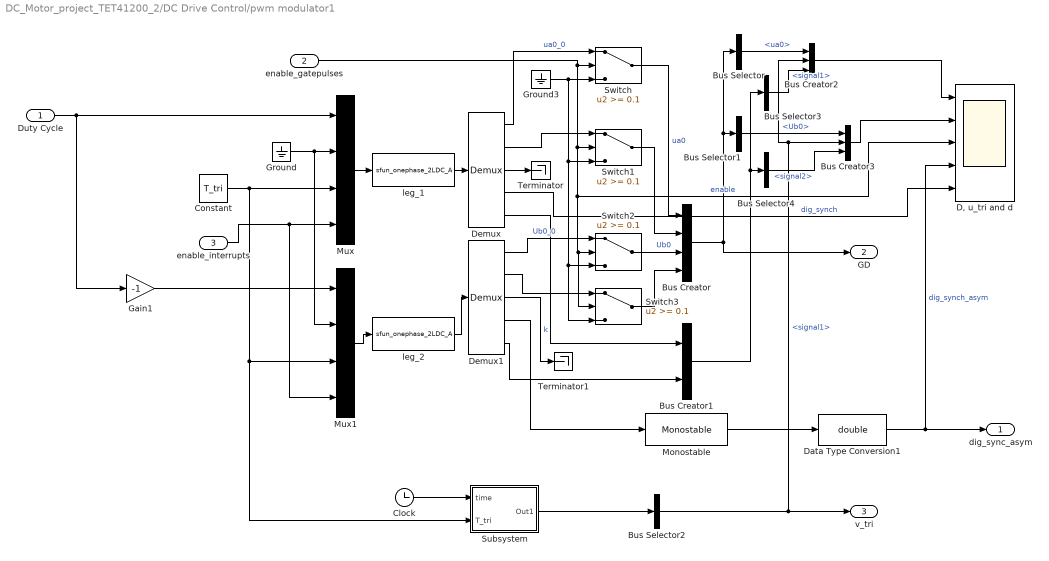
== system DC_Motor_project_TET41200_2/DC Drive Control/pwm modulator1 ==
  Duty Cycle : Inport
  enable_gatepulses : Inport  Port=2
  enable_interrupts : Inport  Port=3
  Bus Creator : BusCreator  Inputs=4
  Bus Creator1 : BusCreator  Inputs=2
  Bus Creator2 : BusCreator  Inputs=3
  Bus Creator3 : BusCreator  Inputs=3
  Bus Selector : BusSelector  OutputSignals=ua0
  Bus Selector1 : BusSelector  OutputSignals=Ub0
  Bus Selector2 : BusSelector  OutputSignals=signal1
  Bus Selector3 : BusSelector  OutputSignals=signal1
  Bus Selector4 : BusSelector  OutputSignals=signal2
  Clock : Clock
  Constant : Constant  Value=T_tri
  "D, u_tri and d " : Scope  NumInputPorts=5
  Data Type Conversion1 : DataTypeConversion  OutDataTypeStr=double  SaturateOnIntegerOverflow=off  RndMeth=Floor
  Demux : Demux  Outputs=5
      settings: DisplayOption=none
  Demux1 : Demux  Outputs=5
      settings: DisplayOption=none
  Gain1 : Gain  Gain=-1
  Ground : Ground
  Ground3 : Ground
  Monostable : spsMonostableLib/Monostable  EdgeDetect=Either  PulseDuration=T_tri/4  ic=0  Ts=0
      settings: LibrarySourceBlock=sps_lib/Control/Monostable
  Mux : Mux
  Mux1 : Mux
  Subsystem : Subsystem
  Switch{,1..3} (4 alike) : Switch  Threshold=0.1  SaturateOnIntegerOverflow=off  InputSameDT=off
  Terminator : Terminator
  Terminator1 : Terminator
  leg_1 : S-Function  FunctionName=sfun_onephase_2LDC_A  Parameters=0,t_dead,t_min,type_signal,asym  SFunctionDeploymentMode=off  EnableBusSupport=off
  leg_2 : S-Function  FunctionName=sfun_onephase_2LDC_A  Parameters=0,t_dead,t_min,type_signal,asym  SFunctionDeploymentMode=off  EnableBusSupport=off
  dig_sync_asym : Outport
  GD : Outport  Port=2
  v_tri : Outport  Port=3
  wires:
  Demux/3 -> Terminator/1
  Constant/1 -> Mux/3, Subsystem/2(T_tri), Mux1/3
  Ground/1 -> Mux1/2, Mux/2
  leg_1/1 -> Demux/1
  leg_2/1 -> Demux1/1
  Mux/1 -> leg_1/1
  Demux/2 -> Switch1/1
  Demux1/5 -> Bus Creator1/2
  Demux/4 -> "D, u_tri and d "/5  "dig_synch"
  Subsystem/1(Out1) -> Bus Selector2/1
  Clock/1 -> Subsystem/1(time)
  Demux/5 -> Bus Creator1/1
  Bus Creator/1 -> GD/1, Bus Selector1/1, Bus Selector/1
  Bus Creator1/1 -> Bus Selector3/1, Bus Selector4/1
  Bus Selector/1 -> Bus Creator2/1  "<ua0>"
  Bus Selector3/1 -> Bus Creator2/3  "<signal1>"
  Bus Selector1/1 -> Bus Creator3/1  "<Ub0>"
  Bus Selector4/1 -> Bus Creator3/3  "<signal2>"
  Bus Creator2/1 -> "D, u_tri and d "/1
  Bus Creator3/1 -> "D, u_tri and d "/2
  Mux1/1 -> leg_2/1
  enable_gatepulses/1 -> Switch/2, Switch3/2, Switch2/2, "D, u_tri and d "/3, Switch1/2  "enable"
  Duty Cycle/1 -> Mux/1, Gain1/1
  Gain1/1 -> Mux1/1
  Switch/1 -> Bus Creator/1  "ua0"
  Demux/1 -> Switch/1  "ua0_0"
  Switch1/1 -> Bus Creator/2
  Ground3/1 -> Switch/3, Switch1/3, Switch2/3, Switch3/3
  Switch2/1 -> Bus Creator/3  "Ub0"
  Switch3/1 -> Bus Creator/4
  Bus Selector2/1 -> Bus Creator2/2, Bus Creator3/2, v_tri/1  "<signal1>"
  Demux1/4 -> Monostable/1
  Monostable/1 -> Data Type Conversion1/1
  Data Type Conversion1/1 -> dig_sync_asym/1, "D, u_tri and d "/4  "dig_synch_asym"
  Demux1/3 -> Terminator1/1  "k"
  enable_interrupts/1 -> Mux1/4, Mux/4
  Demux1/1 -> Switch2/1  "Ub0_0"
  Demux1/2 -> Switch3/1

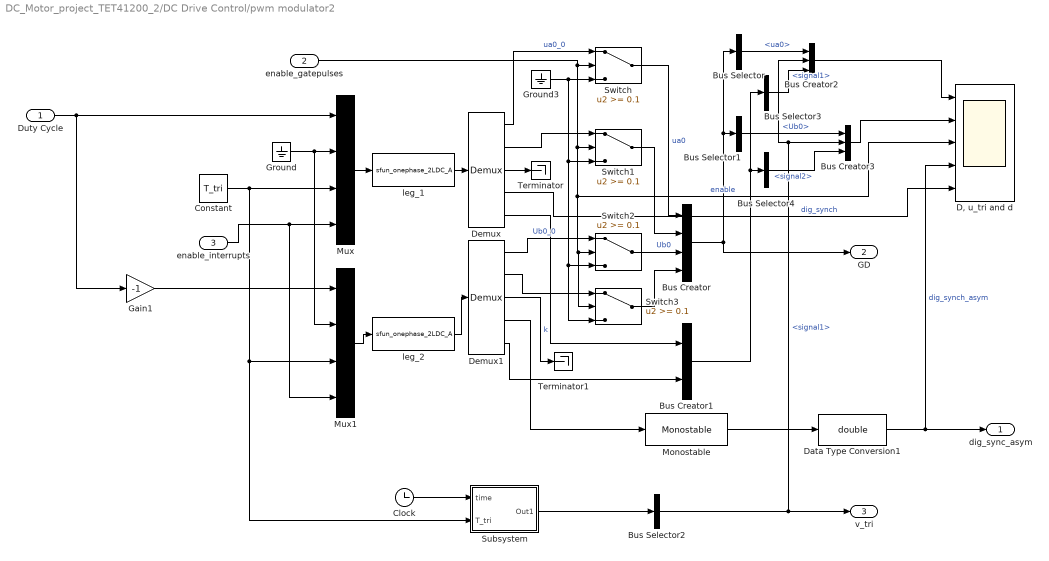
== system DC_Motor_project_TET41200_2/DC Drive Control/pwm modulator2 ==
  Duty Cycle : Inport
  enable_gatepulses : Inport  Port=2
  enable_interrupts : Inport  Port=3
  Bus Creator : BusCreator  Inputs=4
  Bus Creator1 : BusCreator  Inputs=2
  Bus Creator2 : BusCreator  Inputs=3
  Bus Creator3 : BusCreator  Inputs=3
  Bus Selector : BusSelector  OutputSignals=ua0
  Bus Selector1 : BusSelector  OutputSignals=Ub0
  Bus Selector2 : BusSelector  OutputSignals=signal1
  Bus Selector3 : BusSelector  OutputSignals=signal1
  Bus Selector4 : BusSelector  OutputSignals=signal2
  Clock : Clock
  Constant : Constant  Value=T_tri
  "D, u_tri and d " : Scope  NumInputPorts=5
  Data Type Conversion1 : DataTypeConversion  OutDataTypeStr=double  SaturateOnIntegerOverflow=off  RndMeth=Floor
  Demux : Demux  Outputs=5
      settings: DisplayOption=none
  Demux1 : Demux  Outputs=5
      settings: DisplayOption=none
  Gain1 : Gain  Gain=-1
  Ground : Ground
  Ground3 : Ground
  Monostable : spsMonostableLib/Monostable  EdgeDetect=Either  PulseDuration=T_tri/4  ic=0  Ts=0
      settings: LibrarySourceBlock=sps_lib/Control/Monostable
  Mux : Mux
  Mux1 : Mux
  Subsystem : Subsystem
  Switch{,1..3} (4 alike) : Switch  Threshold=0.1  SaturateOnIntegerOverflow=off  InputSameDT=off
  Terminator : Terminator
  Terminator1 : Terminator
  leg_1 : S-Function  FunctionName=sfun_onephase_2LDC_A  Parameters=0,t_dead,t_min,type_signal,asym  SFunctionDeploymentMode=off  EnableBusSupport=off
  leg_2 : S-Function  FunctionName=sfun_onephase_2LDC_A  Parameters=0,t_dead,t_min,type_signal,asym  SFunctionDeploymentMode=off  EnableBusSupport=off
  dig_sync_asym : Outport
  GD : Outport  Port=2
  v_tri : Outport  Port=3
  wires:
  Demux/3 -> Terminator/1
  Constant/1 -> Mux/3, Subsystem/2(T_tri), Mux1/3
  Ground/1 -> Mux1/2, Mux/2
  leg_1/1 -> Demux/1
  leg_2/1 -> Demux1/1
  Mux/1 -> leg_1/1
  Demux/2 -> Switch1/1
  Demux1/5 -> Bus Creator1/2
  Demux/4 -> "D, u_tri and d "/5  "dig_synch"
  Subsystem/1(Out1) -> Bus Selector2/1
  Clock/1 -> Subsystem/1(time)
  Demux/5 -> Bus Creator1/1
  Bus Creator/1 -> GD/1, Bus Selector1/1, Bus Selector/1
  Bus Creator1/1 -> Bus Selector3/1, Bus Selector4/1
  Bus Selector/1 -> Bus Creator2/1  "<ua0>"
  Bus Selector3/1 -> Bus Creator2/3  "<signal1>"
  Bus Selector1/1 -> Bus Creator3/1  "<Ub0>"
  Bus Selector4/1 -> Bus Creator3/3  "<signal2>"
  Bus Creator2/1 -> "D, u_tri and d "/1
  Bus Creator3/1 -> "D, u_tri and d "/2
  Mux1/1 -> leg_2/1
  enable_gatepulses/1 -> Switch/2, Switch3/2, Switch2/2, "D, u_tri and d "/3, Switch1/2  "enable"
  Duty Cycle/1 -> Mux/1, Gain1/1
  Gain1/1 -> Mux1/1
  Switch/1 -> Bus Creator/1  "ua0"
  Demux/1 -> Switch/1  "ua0_0"
  Switch1/1 -> Bus Creator/2
  Ground3/1 -> Switch/3, Switch1/3, Switch2/3, Switch3/3
  Switch2/1 -> Bus Creator/3  "Ub0"
  Switch3/1 -> Bus Creator/4
  Bus Selector2/1 -> Bus Creator2/2, Bus Creator3/2, v_tri/1  "<signal1>"
  Demux1/4 -> Monostable/1
  Monostable/1 -> Data Type Conversion1/1
  Data Type Conversion1/1 -> dig_sync_asym/1, "D, u_tri and d "/4  "dig_synch_asym"
  Demux1/3 -> Terminator1/1  "k"
  enable_interrupts/1 -> Mux1/4, Mux/4
  Demux1/1 -> Switch2/1  "Ub0_0"
  Demux1/2 -> Switch3/1

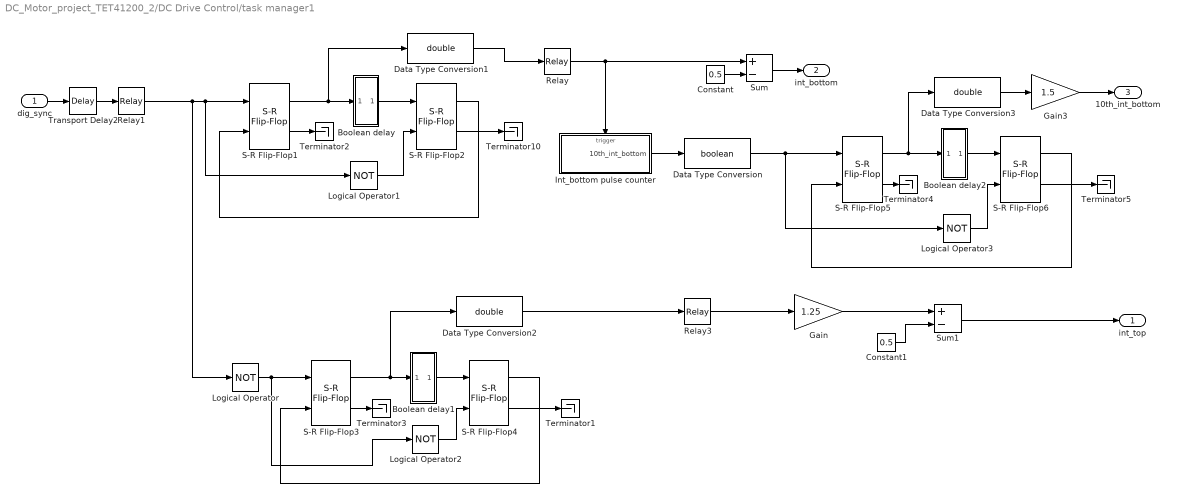
== system DC_Motor_project_TET41200_2/DC Drive Control/task manager1 ==
  dig_sync : Inport
  Boolean delay : Subsystem
  Boolean delay1 : Subsystem
  Boolean delay2 : Subsystem
  Constant : Constant  Value=0.5
  Constant1 : Constant  Value=0.5
  Data Type Conversion : DataTypeConversion  OutDataTypeStr=boolean  SaturateOnIntegerOverflow=off  RndMeth=Floor
  Data Type Conversion1 : DataTypeConversion  OutDataTypeStr=double  SaturateOnIntegerOverflow=off  RndMeth=Floor
  Data Type Conversion2 : DataTypeConversion  OutDataTypeStr=double  SaturateOnIntegerOverflow=off  RndMeth=Floor
  Data Type Conversion3 : DataTypeConversion  OutDataTypeStr=double  SaturateOnIntegerOverflow=off  RndMeth=Floor
  Gain : Gain  Gain=1.25  SaturateOnIntegerOverflow=on  OutDataTypeStr=Inherit: Same as input  ParamDataTypeStr=Inherit: Same as input
  Gain3 : Gain  Gain=1.5  SaturateOnIntegerOverflow=on  OutDataTypeStr=Inherit: Same as input  ParamDataTypeStr=Inherit: Same as input
  Int_bottom pulse counter : Subsystem  TreatAsAtomicUnit=on
  Logical Operator : Logic  Operator=NOT  AllPortsSameDT=off
  Logical Operator1 : Logic  Operator=NOT
  Logical Operator2 : Logic  Operator=NOT
  Logical Operator3 : Logic  Operator=NOT
  Relay : Relay  OnSwitchValue=0.5  OffSwitchValue=0.5-eps
  Relay1 : Relay  OutDataTypeStr=Inherit: Inherit via back propagation
  Relay3 : Relay  OnSwitchValue=0.5  OffSwitchValue=0.5-eps
  S-R Flip-Flop{1..6} (6 alike) : simulink_extras/Flip Flops/S-R Flip-Flop  initial_condition=0
  Sum : Sum  Inputs=+-  InputSameDT=on  SaturateOnIntegerOverflow=on  OutDataTypeStr=Inherit: Same as first input
  Sum1 : Sum  Inputs=+-  InputSameDT=on  SaturateOnIntegerOverflow=on  OutDataTypeStr=Inherit: Same as first input
  Terminator{1..5,10} (6 alike) : Terminator
  Transport Delay2 : TransportDelay  DelayTime=2e-6
  int_top : Outport
  int_bottom : Outport  Port=2
  10th_int_bottom : Outport  Port=3
  wires:
  Data Type Conversion3/1 -> Gain3/1
  Data Type Conversion2/1 -> Relay3/1
  Data Type Conversion1/1 -> Relay/1
  Data Type Conversion/1 -> Logical Operator3/1, S-R Flip-Flop5/1
  Int_bottom pulse counter/1(10th_int_bottom) -> Data Type Conversion/1
  S-R Flip-Flop3/2 -> Terminator3/1
  S-R Flip-Flop1/2 -> Terminator2/1
  S-R Flip-Flop4/2 -> Terminator1/1
  S-R Flip-Flop2/2 -> Terminator10/1
  Gain3/1 -> 10th_int_bottom/1
  S-R Flip-Flop6/2 -> Terminator5/1
  S-R Flip-Flop5/2 -> Terminator4/1
  S-R Flip-Flop5/1 -> Data Type Conversion3/1, Boolean delay2/1(In1)
  Boolean delay2/1(Out1) -> S-R Flip-Flop6/1
  S-R Flip-Flop6/1 -> S-R Flip-Flop5/2
  Logical Operator3/1 -> S-R Flip-Flop6/2
  Sum1/1 -> int_top/1
  Gain/1 -> Sum1/1
  Constant1/1 -> Sum1/2
  Constant/1 -> Sum/2
  Sum/1 -> int_bottom/1
  S-R Flip-Flop1/1 -> Data Type Conversion1/1, Boolean delay/1(In1)
  Boolean delay/1(Out1) -> S-R Flip-Flop2/1
  S-R Flip-Flop2/1 -> S-R Flip-Flop1/2
  Logical Operator1/1 -> S-R Flip-Flop2/2
  Relay/1 -> Int_bottom pulse counter/Trigger, Sum/1
  Logical Operator/1 -> Logical Operator2/1, S-R Flip-Flop3/1
  S-R Flip-Flop3/1 -> Data Type Conversion2/1, Boolean delay1/1(In1)
  Boolean delay1/1(Out1) -> S-R Flip-Flop4/1
  S-R Flip-Flop4/1 -> S-R Flip-Flop3/2
  Logical Operator2/1 -> S-R Flip-Flop4/2
  Relay3/1 -> Gain/1
  Transport Delay2/1 -> Relay1/1
  Relay1/1 -> S-R Flip-Flop1/1, Logical Operator1/1, Logical Operator/1
  dig_sync/1 -> Transport Delay2/1

== system DC_Motor_project_TET41200_2/DC Machine/DC machine ==
  n : Inport
  u_a : Inport  Port=2
  u_f : Inport  Port=3
  Gain1 : Gain  Gain=1/T_f  SaturateOnIntegerOverflow=on  OutDataTypeStr=Inherit: Same as input  ParamDataTypeStr=Inherit: Same as input
  Gain6 : Gain  Gain=1/l_a  SaturateOnIntegerOverflow=on  OutDataTypeStr=Inherit: Same as input  ParamDataTypeStr=Inherit: Same as input
  Product : Product
  Product1 : Product
  Sum1 : Sum  Inputs=|+-  InputSameDT=on  SaturateOnIntegerOverflow=on  OutDataTypeStr=Inherit: Same as first input
  Sum5 : Sum  Inputs=-|+|-  InputSameDT=on  SaturateOnIntegerOverflow=on  OutDataTypeStr=Inherit: Same as first input
  dif/dt : Integrator
  i_a1 : Integrator
  rs * i_a : Gain  Gain=r_a  SaturateOnIntegerOverflow=on  OutDataTypeStr=Inherit: Same as input  ParamDataTypeStr=Inherit: Same as input
  t_e [pu] : Outport
  i_a : Outport  Port=2
  i_f : Outport  Port=3
  wires:
  u_a/1 -> Sum5/2  "u_a"
  i_a1/1 -> Product/1, rs * i_a/1, i_a/1  "i_a"
  Gain6/1 -> i_a1/1
  rs * i_a/1 -> Sum5/1
  Sum5/1 -> Gain6/1
  Product/1 -> t_e [pu]/1
  Product1/1 -> Sum5/3  "e_a"
  dif/dt/1 -> Product1/1, Product/2, Sum1/2, i_f/1  "i_f"
  Gain1/1 -> dif/dt/1
  u_f/1 -> Sum1/1  "u_f"
  Sum1/1 -> Gain1/1
  n/1 -> Product1/2

== system DC_Motor_project_TET41200_2/DCDC chopper/u_m ==
  Ia : Inport
  Bus Creator : BusCreator  Inputs=4
  Voltage Measurement1 : spsVoltageMeasurementLib/Voltage Measurement  PhasorSimulation=off  OutputType=Complex  PSBequivalent=0
  Voltage Measurement2 : spsVoltageMeasurementLib/Voltage Measurement  PhasorSimulation=off  OutputType=Complex  PSBequivalent=0
  Voltage Measurement3 : spsVoltageMeasurementLib/Voltage Measurement  PhasorSimulation=off  OutputType=Complex  PSBequivalent=0
  DC+ : PMIOPort  Side=Left
  DC- : PMIOPort  Port=2  Side=Left
  A : PMIOPort  Port=3  Side=Left
  B : PMIOPort  Port=4  Side=Left
  U : Outport
  wires:
  Ia/1 -> Bus Creator/4  "Iout [A]"
  Voltage Measurement3/1 -> Bus Creator/1  "Udc [V]"
  Voltage Measurement2/1 -> Bus Creator/2  "UA [V]"
  Bus Creator/1 -> U/1
  Voltage Measurement1/1 -> Bus Creator/3  "UB [V]"
  connections:
  DC-/RConn1 -- Voltage Measurement1/LConn2 -- Voltage Measurement3/LConn2 -- Voltage Measurement2/LConn2
  DC+/RConn1 -- Voltage Measurement3/LConn1
  A/RConn1 -- Voltage Measurement2/LConn1
  Voltage Measurement1/LConn1 -- B/RConn1

== system DC_Motor_project_TET41200_2/Field DCDC chopper/u_m ==
  Ia : Inport
  Bus Creator : BusCreator  Inputs=4
  Voltage Measurement1 : spsVoltageMeasurementLib/Voltage Measurement  PhasorSimulation=off  OutputType=Complex  PSBequivalent=0
  Voltage Measurement2 : spsVoltageMeasurementLib/Voltage Measurement  PhasorSimulation=off  OutputType=Complex  PSBequivalent=0
  Voltage Measurement3 : spsVoltageMeasurementLib/Voltage Measurement  PhasorSimulation=off  OutputType=Complex  PSBequivalent=0
  DC+ : PMIOPort  Side=Left
  DC- : PMIOPort  Port=2  Side=Left
  A : PMIOPort  Port=3  Side=Left
  B : PMIOPort  Port=4  Side=Left
  U : Outport
  wires:
  Ia/1 -> Bus Creator/4  "Iout [A]"
  Voltage Measurement3/1 -> Bus Creator/1  "Udc [V]"
  Voltage Measurement2/1 -> Bus Creator/2  "UA [V]"
  Bus Creator/1 -> U/1
  Voltage Measurement1/1 -> Bus Creator/3  "UB [V]"
  connections:
  DC-/RConn1 -- Voltage Measurement1/LConn2 -- Voltage Measurement3/LConn2 -- Voltage Measurement2/LConn2
  DC+/RConn1 -- Voltage Measurement3/LConn1
  A/RConn1 -- Voltage Measurement2/LConn1
  Voltage Measurement1/LConn1 -- B/RConn1

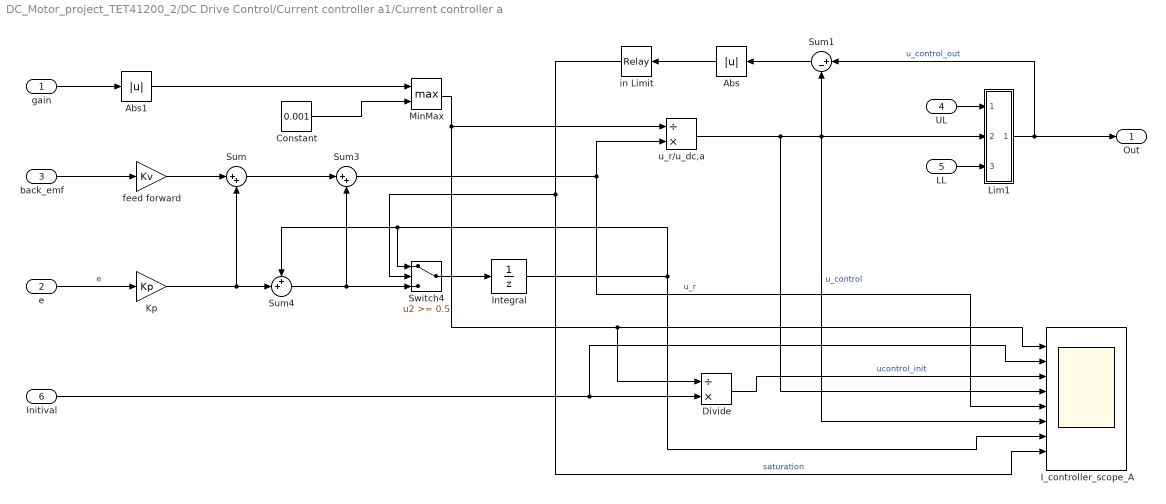
== system DC_Motor_project_TET41200_2/DC Drive Control/Current controller a1/Current controller a ==
  gain : Inport
  e : Inport  Port=2
  back_emf : Inport  Port=3
  UL : Inport  Port=4
  LL : Inport  Port=5
  Initival : Inport  Port=6
  Abs : Abs  SaturateOnIntegerOverflow=off
  Abs1 : Abs  SaturateOnIntegerOverflow=off
  Constant : Constant  Value=0.001
  Divide : Product  Inputs=/*
  I_controller_scope_A : Scope  NumInputPorts=8
  Integral : UnitDelay  SampleTime=-1  HasFrameUpgradeWarning=on
  Kp : Gain  Gain=Kp  SaturateOnIntegerOverflow=on  OutDataTypeStr=Inherit: Same as input  ParamDataTypeStr=Inherit: Same as input
  Lim1 : Subsystem
      mask Display:
      | plot([0.3 0.5 0.7 0.3], [0.1 0.3  0.1 0.1])
      | plot([0.3 0.5 0.7 0.3], [0.9 0.7  0.9 0.9])
  MinMax : MinMax  Function=max  Inputs=2
  Sum : Sum  Inputs=|++  InputSameDT=on  SaturateOnIntegerOverflow=on  OutDataTypeStr=Inherit: Same as first input
  Sum1 : Sum  Inputs=|+-  InputSameDT=on  SaturateOnIntegerOverflow=on  OutDataTypeStr=Inherit: Same as first input
  Sum3 : Sum  Inputs=|++  InputSameDT=on  SaturateOnIntegerOverflow=on  OutDataTypeStr=Inherit: Same as first input
  Sum4 : Sum  Inputs=++|  InputSameDT=on  SaturateOnIntegerOverflow=on  OutDataTypeStr=Inherit: Same as first input
  Switch4 : Switch  Threshold=0.5
  feed forward : Gain  Gain=Kv  SaturateOnIntegerOverflow=on  OutDataTypeStr=Inherit: Same as input  ParamDataTypeStr=Inherit: Same as input
  in Limit : Relay  OffSwitchValue=0
  u_r/u_dc,a : Product  Inputs=/*
  Out : Outport
  wires:
  u_r/u_dc,a/1 -> I_controller_scope_A/6, Lim1/2(In), Sum1/2, I_controller_scope_A/4  "u_control"
  e/1 -> Kp/1  "e"
  Divide/1 -> I_controller_scope_A/3  "ucontrol_init"
  feed forward/1 -> Sum/1
  Kp/1 -> Sum4/2, Sum/2
  back_emf/1 -> feed forward/1
  UL/1 -> Lim1/1(UL)
  Lim1/1(Out) -> Out/1, Sum1/1  "u_control_out"
  Sum/1 -> Sum3/1
  Sum4/1 -> Switch4/3, Sum3/2
  Integral/1 -> Sum4/1, Switch4/1, I_controller_scope_A/7
  Sum3/1 -> u_r/u_dc,a/2, I_controller_scope_A/5  "u_r"
  LL/1 -> Lim1/3(LL)
  Abs/1 -> in Limit/1
  Sum1/1 -> Abs/1
  in Limit/1 -> Switch4/2, I_controller_scope_A/8  "saturation"
  Switch4/1 -> Integral/1
  Initival/1 -> I_controller_scope_A/2, Divide/2
  MinMax/1 -> Divide/1, I_controller_scope_A/1, u_r/u_dc,a/1
  Constant/1 -> MinMax/2
  gain/1 -> Abs1/1
  Abs1/1 -> MinMax/1

== system DC_Motor_project_TET41200_2/DC Drive Control/Current controller a2/Current controller f ==
  gain : Inport
  e : Inport  Port=2
  UL : Inport  Port=3
  LL : Inport  Port=4
  Abs : Abs  SaturateOnIntegerOverflow=off
  Abs1 : Abs  SaturateOnIntegerOverflow=off
  Anti windup relay : Relay  OffSwitchValue=0
  Constant : Constant  Value=0.001
  I_controller_scope_A : Scope  NumInputPorts=5
  Integral : UnitDelay  SampleTime=-1  HasFrameUpgradeWarning=on
  Kp : Gain  Gain=Kp  SaturateOnIntegerOverflow=on  OutDataTypeStr=Inherit: Same as input  ParamDataTypeStr=Inherit: Same as input
  Limitation block : Subsystem
      mask Display:
      | plot([0.3 0.5 0.7 0.3], [0.1 0.3  0.1 0.1])
      | plot([0.3 0.5 0.7 0.3], [0.9 0.7  0.9 0.9])
  MinMax : MinMax  Function=max  Inputs=2
  Sum1 : Sum  Inputs=|+-  InputSameDT=on  SaturateOnIntegerOverflow=on  OutDataTypeStr=Inherit: Same as first input
  Sum4 : Sum  Inputs=++|  InputSameDT=on  SaturateOnIntegerOverflow=on  OutDataTypeStr=Inherit: Same as first input
  Switch4 : Switch  Threshold=0.5
  u_r/u_dc(pu) : Product  Inputs=/*
  Out : Outport
  wires:
  u_r/u_dc(pu)/1 -> Limitation block/2(In), I_controller_scope_A/3, Sum1/2  "u_control"
  e/1 -> Kp/1  "e"
  Kp/1 -> Sum4/2
  UL/1 -> Limitation block/1(UL)
  Limitation block/1(Out) -> Sum1/1, Out/1  "u_control_limit"
  Integral/1 -> Switch4/1, Sum4/1, I_controller_scope_A/4  "integral"
  Sum4/1 -> Switch4/3, u_r/u_dc(pu)/2, I_controller_scope_A/2  "u_r"
  LL/1 -> Limitation block/3(LL)
  Abs/1 -> Anti windup relay/1
  Sum1/1 -> Abs/1
  Anti windup relay/1 -> I_controller_scope_A/5, Switch4/2  "saturation"
  Switch4/1 -> Integral/1
  MinMax/1 -> I_controller_scope_A/1, u_r/u_dc(pu)/1  "u_dc"
  Constant/1 -> MinMax/2
  gain/1 -> Abs1/1
  Abs1/1 -> MinMax/1
